simulink model "dos_masas_rotacional"  (R2018a)
settings: Solver=VariableStepAuto  StartTime=0.0  StopTime=12  RelTol=1e-3
InitFcn:
  | J1 = 5
  | J2 = 4
  | K1 = 10
  | K2 = 8
  | T = 1
settings Model: Creator=Arturo  LastModifiedBy=Arturo

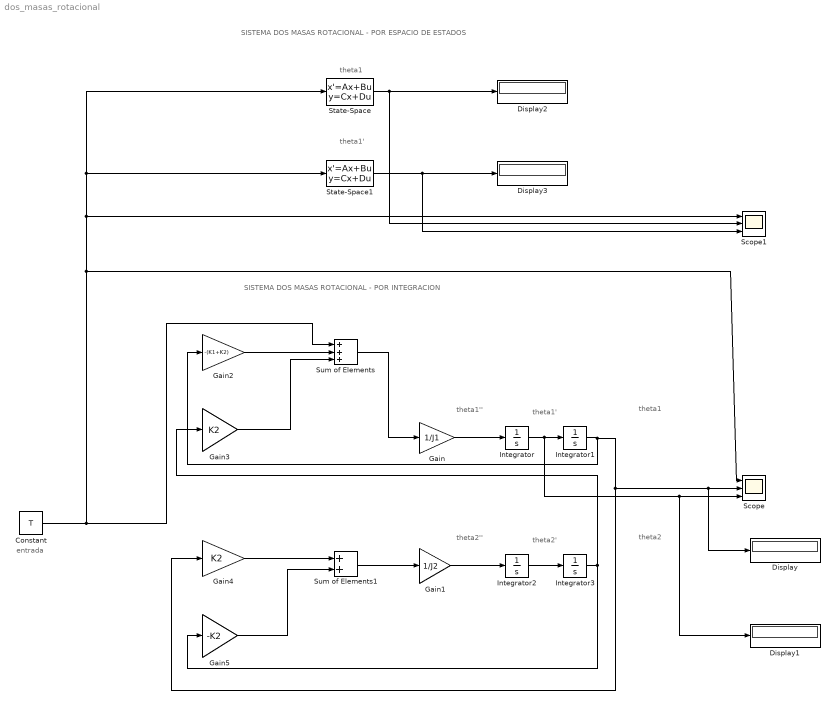
== system dos_masas_rotacional ==
  note: entrada
  note: SISTEMA DOS MASAS ROTACIONAL - POR ESPACIO DE ESTADOS
  note: SISTEMA DOS MASAS ROTACIONAL - POR INTEGRACION
  note: theta1
  note: theta1''
  note: theta1'
  note: theta2'
  note: theta2
  note: theta2''
  note: theta1
  note: theta1'
  Constant : Constant  Value=T
  Display{,1..3} (4 alike) : Display
  Gain : Gain  Gain=1/J1
  Gain1 : Gain  Gain=1/J2
  Gain2 : Gain  Gain=-(K1+K2)
  Gain3 : Gain  Gain=K2
  Gain4 : Gain  Gain=K2
  Gain5 : Gain  Gain=-K2
  Integrator{,1..3} (4 alike) : Integrator
  Scope : Scope  NumInputPorts=3
  Scope1 : Scope  NumInputPorts=3
  State-Space : StateSpace  A=[0 1 0 0; -((K1+K2)/J1) 0 K2/J1 0; 0 0 0 1; K2/J2 0 -K2/J2 0]  B=[0; 1/J1; 0; 0]  C=[1 0 0 0]  D=0  InitialCondition=0
  State-Space1 : StateSpace  A=[0 1 0 0; -((K1+K2)/J1) 0 K2/J1 0; 0 0 0 1; K2/J2 0 -K2/J2 0]  B=[0; 1/J1; 0; 0]  C=[0 1 0 0]  D=0  InitialCondition=0
  Sum of Elements : Sum  Inputs=3
  Sum of Elements1 : Sum  Inputs=2
  wires:
  Integrator/1 -> Display1/1, Scope/3, Integrator1/1
  Integrator2/1 -> Integrator3/1
  Integrator1/1 -> Display/1, Scope/2, Gain4/1, Gain2/1
  Gain2/1 -> Sum of Elements/2
  Integrator3/1 -> Gain5/1, Gain3/1
  Gain3/1 -> Sum of Elements/3
  Constant/1 -> Scope/1, Scope1/1, State-Space1/1, State-Space/1, Sum of Elements/1
  Sum of Elements/1 -> Gain/1
  Gain/1 -> Integrator/1
  Gain5/1 -> Sum of Elements1/2
  Gain4/1 -> Sum of Elements1/1
  Sum of Elements1/1 -> Gain1/1
  Gain1/1 -> Integrator2/1
  State-Space/1 -> Scope1/2, Display2/1
  State-Space1/1 -> Scope1/3, Display3/1
